simulink model "Wind1500KW_bilbil_finished"  (R2020a)
settings: Solver=VariableStepAuto  StartTime=0.0  StopTime=20  RelTol=1e-3
libraries: powerlib x12, powerlib_meascontrol x10, simulink x7
settings Model: Creator=Administrator  LastModifiedBy=Administrator

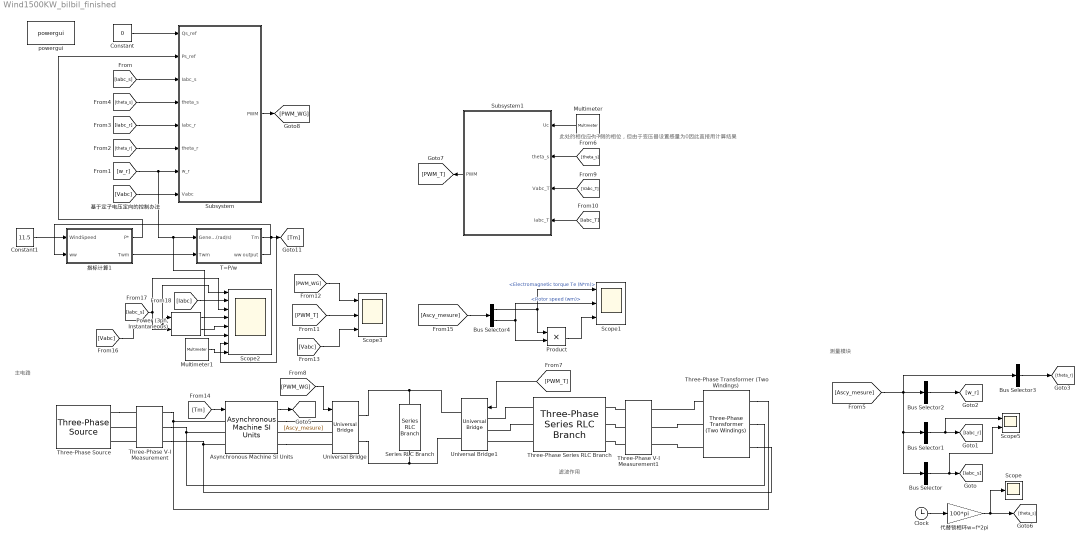
== system Wind1500KW_bilbil_finished ==
  note: 滤波作用
  note: 此处的相位应为T侧的相位，但由于变压器设置感量为0因此直接用计算结果
  note: 测量模块
  note: 主电路
  Asynchronous Machine SI Units : powerlib/Machines/Asynchronous Machine SI Units  RotorType=Wound  PresetModel=No  MechanicalLoad=Torque Tm  ShowDetailedParameters=on  ReferenceFrame=Rotor  Units=SI  MeasurementBus=off  NominalParameters=[1.5e+06 690 50]  Stator=[0.0055 1.56e-4]  Rotor=[0.00621 2.26e-04]  Cage1=[0.4155 0.002066]  Cage2=[0.4168 0.0003495]  Lm=0.01101  Mechanical=[30 0.005879 2]  PolePairs=2  InitialConditions=[0 0 0 0 0 0 0 0]  SimulateSaturation=off  Saturation=[14.03593122, 27.81365428, 53.79336849, 72.68890987, 97.98006896, 148.6815601, 215.7428561, 302.9841135, 428.7778367 ; 230, 322, 414, 460, 506, 552, 598, 644, 690]  LoadFlowParameters=1492000  TsPowergui=0  TsBlock=-1  IterativeModel=Trapezoidal non iterative  IterativeDiscreteModel=Trapezoidal non iterative  Pmec=1.492e+006
  Bus Selector : BusSelector  OutputSignals=Stator measurements.Stator current is_a (A),Stator measurements.Stator current is_b (A),Stator measurements.Stator current is_c (A)  OutputAsBus=on
  Bus Selector1 : BusSelector  OutputSignals=Rotor measurements.Rotor current ir_a (A),Rotor measurements.Rotor current ir_b (A),Rotor measurements.Rotor current ir_c (A)  OutputAsBus=on
  Bus Selector2 : BusSelector  OutputSignals=Mechanical.Rotor speed (wm)  OutputAsBus=on
  Bus Selector3 : BusSelector  OutputSignals=Mechanical.Rotor angle thetam (rad)  OutputAsBus=on
  Bus Selector4 : BusSelector  OutputSignals=Mechanical.Electromagnetic torque Te (N*m),Mechanical.Rotor speed (wm)
  Clock : Clock
  Constant : Constant  Value=0
  Constant1 : Constant  Value=11.5
  Multimeter : powerlib/Measurements/Multimeter  PhasorSimulation=off  OutputType=Complex  sel=1  L=1  Gain=1  yselected={'Ub: Series RLC Branch'};  PSBOutputType=1  PSBequivalent=0  AxesSetting=[0,0.1,-100,100]  Display=0  SavedBlockNames=-11
  Multimeter1 : powerlib/Measurements/Multimeter  PhasorSimulation=off  OutputType=Complex  sel=1  L=1  Gain=1  yselected={'Ub: Series RLC Branch'};  PSBOutputType=1  PSBequivalent=0  AxesSetting=[0,0.1,-100,100]  Display=0  SavedBlockNames=-11
  "Power (3ph, Instantaneous)" : powerlib_meascontrol/Measurements/Power (3ph, Instantaneous)
  Product : Product
  Scope : Scope
  Scope1 : Scope  NumInputPorts=3
  Scope2 : Scope  NumInputPorts=8
  Scope3 : Scope  NumInputPorts=3
  Scope5 : Scope  NumInputPorts=2
  Series RLC Branch : powerlib/Elements/Series RLC Branch  LConnTagsString=__new0  RConnTagsString=__new0  BranchType=C  Resistance=1  Inductance=1e-3  SetiL0=off  InitialCurrent=0  Capacitance=1e-2  Setx0=off  InitialVoltage=1200  Measurements=Branch voltage
  Subsystem : Subsystem
  Subsystem1 : Subsystem
  T=P/w : Subsystem
  Three-Phase Series RLC Branch : powerlib/Elements/Three-Phase Series RLC Branch  LConnTagsString=A|B|C  RConnTagsString=A|B|C  BranchType=RL  Resistance=0.05  Inductance=1.2e-2  Capacitance=1e-6  Measurements=None
  Three-Phase Transformer (Two Windings) : powerlib/Elements/Three-Phase Transformer (Two Windings)  Winding1Connection=Yg  Winding2Connection=Yg  CoreType=Three single-phase transformers  SetSaturation=off  Hysteresis=off  DataFile='hysteresis'  SetInitialFlux=off  Measurements=None  UNITS=SI  NominalPower=[ 1e6 , 50 ]  Winding1=[890 0.001 0]  Winding2=[690 0.001 0]  Rm=1.0805e+03  Lm=4  L0=0.5  Saturation=[0 0;0.66653 1910.3;277.72 2419.7]  InitialFluxes=[ 0.8 , -0.8 , 0.7 ]  BreakLoop=off  DiscreteSolver=Backward Euler robust  DataType=on  TransfoNumber=1
  Three-Phase V-I Measurement : powerlib/Measurements/Three-Phase V-I Measurement  VoltageMeasurement=phase-to-ground  SetLabelV=on  LabelV=Vabc  Vpu=off  VpuLL=off  CurrentMeasurement=yes  SetLabelI=on  LabelI=Iabc  Ipu=off  Pbase=100e6  Vbase=500e3  OutputType=Complex  PhasorSimulation=off  PSBequivalent=0
  Three-Phase V-I Measurement1 : powerlib/Measurements/Three-Phase V-I Measurement  VoltageMeasurement=phase-to-ground  SetLabelV=on  LabelV=Vabc_T  Vpu=off  VpuLL=off  CurrentMeasurement=yes  SetLabelI=on  LabelI=Iabc_T  Ipu=off  Pbase=100e6  Vbase=500e3  OutputType=Complex  PhasorSimulation=off  PSBequivalent=0
  Three-Phase Source : powerlib/Electrical Sources/Three-Phase Source  InternalConnection=Yg  VoltagePhases=off  Voltage=690  PhaseAngle=0  Voltage_phases=[25e3 25e3 25e3]/sqrt(3)  PhaseAngles_phases=[0 -120 +120]  Frequency=50  NonIdealSource=off  SpecifyImpedance=off  Resistance=0.8929  Inductance=16.58e-3  ShortCircuitLevel=100e6  BaseVoltage=690  XRratio=7  BusType=swing  Pref=10e3  Qref=0  Prefabc=[10e3, 10e3, 10e3]  Qrefabc=[0, 0, 0]  Qmin=-inf  Qmax=inf
  Universal Bridge : powerlib/Power Electronics/Universal Bridge  Arms=3  SnubberResistance=1e5  SnubberCapacitance=inf  Device=MOSFET / Diodes  Ron=1e-3  Lon=0  ForwardVoltages="[  0  0  ]"  ForwardVoltage=0  GTOparameters=[ 10e-6 , 20e-6 ]  IGBTparameters=[ 1e-6 , 2e-6 ]  Measurements=None  Measurements_2=None  converterType=Rectifier
  Universal Bridge1 : powerlib/Power Electronics/Universal Bridge  Arms=3  SnubberResistance=1e5  SnubberCapacitance=inf  Device=MOSFET / Diodes  Ron=1e-3  Lon=0  ForwardVoltages="[  0  0  ]"  ForwardVoltage=0  GTOparameters=[ 10e-6 , 20e-6 ]  IGBTparameters=[ 1e-6 , 2e-6 ]  Measurements=None  Measurements_2=None  converterType=Rectifier
  powergui : powerlib/powergui  Priority=1  SimulationMode=Discrete  SampleTime=5e-6  frequency=60  Iterations=50  frequencyindice=50  Pbase=100e6  ErrMax=1e-4  UnitsV=kV  UnitsW=MW  buscounter=0  FunctionMessages=off  echomessages=off  EnableUseOfTLC=off  CurrentSourceSwitches=off  DisableSnubberDevices=off  DisableRonSwitches=off  DisableVfSwitches=off  DisplayEquations=off  AutomaticDiscreteSolvers=off  SolverType=Tustin/Backward Euler (TBE)  Interpol=off  ExternalGateDelay=off  methode=off  Ts=100  x0status=blocks  SPID=on  SwTol=0  HookPort=off  NonlinearTolerance=1e-4  nMaxIteration=100  ContinueOnMaxIteration=off  RestoreLinks=warning  ResistiveCurrentMeasurement=off  Frange=[0:2:500]  Ylog=off  Xlog=on  ShowGrid=off  save=off  variable=ZData  structure=0  ZoomFFT=off  StartTime=0.0  cycles=1  DisplayStyle=1  fundamental=60  FreqAxis=off  MaxFrequency=1000  frequencyindicesteady=1  RmsSteady=1  display=off
  代替锁相环w=f*2pi : Gain  Gain=100*pi
  指标计算1 : Subsystem
  wires:
  指标计算1/2(Twm) -> T=P/w/2(Twm)
  T=P/w/2(ww output) -> 指标计算1/2(ww)
  Clock/1 -> 代替锁相环w=f*2pi/1
  代替锁相环w=f*2pi/1 -> [theta_s], Scope/1
  Bus Selector/1 -> Scope5/2, [Iabc_s]
  Bus Selector1/1 -> Scope5/1, [Iabc_r]
  Bus Selector2/1 -> [w_r]
  Bus Selector3/1 -> [theta_r]
  Bus Selector4/1 -> Product/1, Scope1/1  "<Electromagnetic torque Te (N*m)>"
  Product/1 -> Scope1/3
  Bus Selector4/2 -> Scope1/2, Product/2  "<Rotor speed (wm)>"
  指标计算1/1(P*) -> Subsystem/2(Ps_ref)
  Constant/1 -> Subsystem/1(Qs_ref)
  [Iabc_s] -> Subsystem/3(Iabc_s)
  [w_r] -> Subsystem/7(w_r), Scope2/6, T=P/w/1(Generator Speed(rad/s))
  [theta_r] -> Subsystem/6(theta_r)
  [Iabc_r] -> Subsystem/5(Iabc_r)
  Constant1/1 -> 指标计算1/1(WindSpeed)
  [Vabc] -> Subsystem/8(Vabc)
  Asynchronous Machine SI Units/1 -> [Ascy_mesure]
  [Ascy_mesure] -> Bus Selector3/1, Bus Selector1/1, Bus Selector/1, Bus Selector2/1
  [theta_s] -> Subsystem/4(theta_s)
  [theta_s] -> Subsystem1/2(theta_s)
  Multimeter/1 -> Subsystem1/1(Uc)
  Subsystem1/1(PWM) -> [PWM_T]
  [PWM_T] -> Universal Bridge1/1
  Subsystem/1(PWM) -> [PWM_WG]
  [PWM_WG] -> Universal Bridge/1
  [Vabc] -> Scope3/3
  [PWM_T] -> Scope3/2
  [PWM_WG] -> Scope3/1
  [Vabc_T] -> Subsystem1/3(Vabc_T)
  [Iabc_T] -> Subsystem1/4(Iabc_T)
  T=P/w/1(Tm) -> Scope2/7, [Tm]
  [Tm] -> Asynchronous Machine SI Units/1
  [Vabc] -> Scope2/1, "Power (3ph, Instantaneous)"/1
  [Iabc_s] -> "Power (3ph, Instantaneous)"/2, Scope2/3
  "Power (3ph, Instantaneous)"/1 -> Scope2/4
  "Power (3ph, Instantaneous)"/2 -> Scope2/5
  [Iabc] -> Scope2/2
  Multimeter1/1 -> Scope2/8
  [Ascy_mesure] -> Bus Selector4/1
  connections:
  Three-Phase Source/RConn1 -- Three-Phase V-I Measurement/LConn1
  Three-Phase V-I Measurement/LConn2 -- Three-Phase Source/RConn2
  Three-Phase V-I Measurement/RConn1 -- Three-Phase Transformer (Two Windings)/RConn1 -- Asynchronous Machine SI Units/LConn1
  Three-Phase V-I Measurement/RConn2 -- Three-Phase Transformer (Two Windings)/RConn2 -- Asynchronous Machine SI Units/LConn2
  Three-Phase V-I Measurement/RConn3 -- Three-Phase Transformer (Two Windings)/RConn3 -- Asynchronous Machine SI Units/LConn3
  Three-Phase V-I Measurement/LConn3 -- Three-Phase Source/RConn3
  Universal Bridge/LConn2 -- Asynchronous Machine SI Units/RConn2
  Asynchronous Machine SI Units/RConn1 -- Universal Bridge/LConn1
  Asynchronous Machine SI Units/RConn3 -- Universal Bridge/LConn3
  Universal Bridge/RConn1 -- Universal Bridge1/RConn1 -- Series RLC Branch/LConn1
  Universal Bridge/RConn2 -- Series RLC Branch/RConn1 -- Universal Bridge1/RConn2
  Three-Phase Series RLC Branch/LConn1 -- Universal Bridge1/LConn1
  Three-Phase Series RLC Branch/LConn2 -- Universal Bridge1/LConn2
  Three-Phase Series RLC Branch/LConn3 -- Universal Bridge1/LConn3
  Three-Phase V-I Measurement1/LConn1 -- Three-Phase Series RLC Branch/RConn1
  Three-Phase V-I Measurement1/LConn2 -- Three-Phase Series RLC Branch/RConn2
  Three-Phase V-I Measurement1/LConn3 -- Three-Phase Series RLC Branch/RConn3
  Three-Phase Transformer (Two Windings)/LConn2 -- Three-Phase V-I Measurement1/RConn2
  Three-Phase Transformer (Two Windings)/LConn1 -- Three-Phase V-I Measurement1/RConn1
  Three-Phase Transformer (Two Windings)/LConn3 -- Three-Phase V-I Measurement1/RConn3

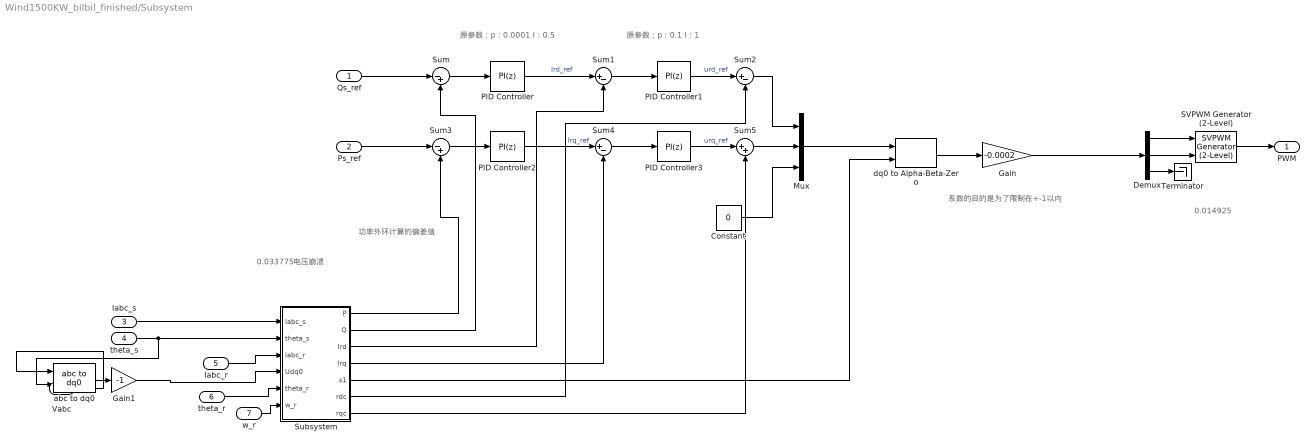
== system Wind1500KW_bilbil_finished/Subsystem ==
  note: 原参数：p：0.0001 I：0.5
  note: 0.033775电压崩溃
  note: 0.014925
  note: 系数的目的是为了限制在+-1以内
  note: 功率外环计算的偏差值
  note: 原参数：p：0.1 I：1
  Qs_ref : Inport
  Ps_ref : Inport  Port=2
  Iabc_s : Inport  Port=3
  theta_s : Inport  Port=4
  Iabc_r : Inport  Port=5
  theta_r : Inport  Port=6
  w_r : Inport  Port=7
  Vabc : Inport  Port=8
  Constant : Constant  Value=0
  Demux : Demux  Outputs=3
  Gain : Gain  Gain=-0.0002
  Gain1 : Gain  Gain=-1
  Mux : Mux  Inputs=3
  PID Controller : simulink/Continuous/PID Controller  Controller=PI  Form=Parallel  TimeDomain=Discrete-time  UseExternalTs=off  SampleTime=5e-6  IntegratorMethod=Forward Euler  FilterMethod=Forward Euler  ControllerParametersSource=internal  P=0.0001  I=0.5  D=0  UseFilter=on  N=100  TunerSelectOption=Transfer Function Based (PID Tuner App)  InitialConditionSource=internal  InitialConditionForIntegrator=0  InitialConditionForFilter=0  DifferentiatorICPrevScaledInput=0  ExternalReset=none  TrackingMode=off  Kt=1  LimitOutput=off  UpperSaturationLimit=inf  LowerSaturationLimit=-inf  LinearizeAsGain=on  AntiWindupMode=none  Kb=1  POutMin=[]  POutMax=[]  IOutMin=[]  IOutMax=[]  DOutMin=[]  DOutMax=[]  NOutMin=[]  NOutMax=[]  SumOutMin=[]  SumOutMax=[]  SaturationOutMin=[]  SaturationOutMax=[]  PParamMin=[]  PParamMax=[]  IParamMin=[]  IParamMax=[]  DParamMin=[]  DParamMax=[]  NParamMin=[]  NParamMax=[]  KbParamMin=[]  KbParamMax=[]  KtParamMin=[]  KtParamMax=[]  KbOutMin=[]  KbOutMax=[]  KtOutMin=[]  KtOutMax=[]  IntegratorOutMin=[]  IntegratorOutMax=[]  FilterOutMin=[]  FilterOutMax=[]  SumI1OutMin=[]  SumI1OutMax=[]  SumI2OutMin=[]  SumI2OutMax=[]  SumI3OutMin=[]  SumI3OutMax=[]  SumI4OutMin=[]  SumI4OutMax=[]  SumDOutMin=[]  SumDOutMax=[]  DifferentiatorOutMin=[]  DifferentiatorOutMax=[]  FilterDiffOutCoefMin=[]  FilterDiffOutCoefMax=[]  ReciprocalOutMin=[]  ReciprocalOutMax=[]  SumDenOutMin=[]  SumDenOutMax=[]  SumNumOutMin=[]  SumNumOutMax=[]  DivideOutMin=[]  DivideOutMax=[]  UdiffTsProdOutMin=[]  UdiffTsProdOutMax=[]  NTsProdOutMin=[]  NTsProdOutMax=[]  UintegralTsProdOutMin=[]  UintegralTsProdOutMax=[]  UngainTsProdOutMin=[]  UngainTsProdOutMax=[]  IntegratorContinuousStateAttributes=''  IntegratorStateMustResolveToSignalObject=off  IntegratorRTWStateStorageClass=Auto  FilterContinuousStateAttributes=''  FilterStateMustResolveToSignalObject=off  FilterRTWStateStorageClass=Auto  ParallelPVariant=InternalParameters  IdealPVariant=Disabled  IVariant=InternalParameters  DVariant=Disabled  IntegratorVariant=Discrete  SatVariant=Disabled  AWVariant=Passthrough  PCopyVariant=Disabled  TRVariant=Disabled  FdbkBlocksVariant=Forward  IdealPFdbkVariant=Disabled  SatFdbkVariant=Disabled  DerivativeFilterVariant=Disabled  NVariant=Disabled  NCopyVariant=Disabled_SignalSpec  FilterICVariant=Disabled  IntegratorICVariant=InternalICs  ExternalResetVariant=Disabled  TRSumVariant=Passthrough  SumFdbkVariant=Disabled  SumVariant=Sum_PI  TsampFilterVariant=InternalTs  TsampNgainVariant=Passthrough  TsampIntegralVariant=Passthrough
  PID Controller1 : simulink/Continuous/PID Controller  Controller=PI  Form=Parallel  TimeDomain=Discrete-time  UseExternalTs=off  SampleTime=5e-6  IntegratorMethod=Forward Euler  FilterMethod=Forward Euler  ControllerParametersSource=internal  P=0.1  I=1.3  D=0  UseFilter=on  N=100  TunerSelectOption=Transfer Function Based (PID Tuner App)  InitialConditionSource=internal  InitialConditionForIntegrator=0  InitialConditionForFilter=0  DifferentiatorICPrevScaledInput=0  ExternalReset=none  TrackingMode=off  Kt=1  LimitOutput=off  UpperSaturationLimit=inf  LowerSaturationLimit=-inf  LinearizeAsGain=on  AntiWindupMode=none  Kb=1  POutMin=[]  POutMax=[]  IOutMin=[]  IOutMax=[]  DOutMin=[]  DOutMax=[]  NOutMin=[]  NOutMax=[]  SumOutMin=[]  SumOutMax=[]  SaturationOutMin=[]  SaturationOutMax=[]  PParamMin=[]  PParamMax=[]  IParamMin=[]  IParamMax=[]  DParamMin=[]  DParamMax=[]  NParamMin=[]  NParamMax=[]  KbParamMin=[]  KbParamMax=[]  KtParamMin=[]  KtParamMax=[]  KbOutMin=[]  KbOutMax=[]  KtOutMin=[]  KtOutMax=[]  IntegratorOutMin=[]  IntegratorOutMax=[]  FilterOutMin=[]  FilterOutMax=[]  SumI1OutMin=[]  SumI1OutMax=[]  SumI2OutMin=[]  SumI2OutMax=[]  SumI3OutMin=[]  SumI3OutMax=[]  SumI4OutMin=[]  SumI4OutMax=[]  SumDOutMin=[]  SumDOutMax=[]  DifferentiatorOutMin=[]  DifferentiatorOutMax=[]  FilterDiffOutCoefMin=[]  FilterDiffOutCoefMax=[]  ReciprocalOutMin=[]  ReciprocalOutMax=[]  SumDenOutMin=[]  SumDenOutMax=[]  SumNumOutMin=[]  SumNumOutMax=[]  DivideOutMin=[]  DivideOutMax=[]  UdiffTsProdOutMin=[]  UdiffTsProdOutMax=[]  NTsProdOutMin=[]  NTsProdOutMax=[]  UintegralTsProdOutMin=[]  UintegralTsProdOutMax=[]  UngainTsProdOutMin=[]  UngainTsProdOutMax=[]  IntegratorContinuousStateAttributes=''  IntegratorStateMustResolveToSignalObject=off  IntegratorRTWStateStorageClass=Auto  FilterContinuousStateAttributes=''  FilterStateMustResolveToSignalObject=off  FilterRTWStateStorageClass=Auto  ParallelPVariant=InternalParameters  IdealPVariant=Disabled  IVariant=InternalParameters  DVariant=Disabled  IntegratorVariant=Discrete  SatVariant=Disabled  AWVariant=Passthrough  PCopyVariant=Disabled  TRVariant=Disabled  FdbkBlocksVariant=Forward  IdealPFdbkVariant=Disabled  SatFdbkVariant=Disabled  DerivativeFilterVariant=Disabled  NVariant=Disabled  NCopyVariant=Disabled_SignalSpec  FilterICVariant=Disabled  IntegratorICVariant=InternalICs  ExternalResetVariant=Disabled  TRSumVariant=Passthrough  SumFdbkVariant=Disabled  SumVariant=Sum_PI  TsampFilterVariant=InternalTs  TsampNgainVariant=Passthrough  TsampIntegralVariant=Passthrough
  PID Controller2 : simulink/Continuous/PID Controller  Controller=PI  Form=Parallel  TimeDomain=Discrete-time  UseExternalTs=off  SampleTime=5e-6  IntegratorMethod=Forward Euler  FilterMethod=Forward Euler  ControllerParametersSource=internal  P=0.0001  I=0.5  D=0  UseFilter=on  N=100  TunerSelectOption=Transfer Function Based (PID Tuner App)  InitialConditionSource=internal  InitialConditionForIntegrator=0  InitialConditionForFilter=0  DifferentiatorICPrevScaledInput=0  ExternalReset=none  TrackingMode=off  Kt=1  LimitOutput=off  UpperSaturationLimit=inf  LowerSaturationLimit=-inf  LinearizeAsGain=on  AntiWindupMode=none  Kb=1  POutMin=[]  POutMax=[]  IOutMin=[]  IOutMax=[]  DOutMin=[]  DOutMax=[]  NOutMin=[]  NOutMax=[]  SumOutMin=[]  SumOutMax=[]  SaturationOutMin=[]  SaturationOutMax=[]  PParamMin=[]  PParamMax=[]  IParamMin=[]  IParamMax=[]  DParamMin=[]  DParamMax=[]  NParamMin=[]  NParamMax=[]  KbParamMin=[]  KbParamMax=[]  KtParamMin=[]  KtParamMax=[]  KbOutMin=[]  KbOutMax=[]  KtOutMin=[]  KtOutMax=[]  IntegratorOutMin=[]  IntegratorOutMax=[]  FilterOutMin=[]  FilterOutMax=[]  SumI1OutMin=[]  SumI1OutMax=[]  SumI2OutMin=[]  SumI2OutMax=[]  SumI3OutMin=[]  SumI3OutMax=[]  SumI4OutMin=[]  SumI4OutMax=[]  SumDOutMin=[]  SumDOutMax=[]  DifferentiatorOutMin=[]  DifferentiatorOutMax=[]  FilterDiffOutCoefMin=[]  FilterDiffOutCoefMax=[]  ReciprocalOutMin=[]  ReciprocalOutMax=[]  SumDenOutMin=[]  SumDenOutMax=[]  SumNumOutMin=[]  SumNumOutMax=[]  DivideOutMin=[]  DivideOutMax=[]  UdiffTsProdOutMin=[]  UdiffTsProdOutMax=[]  NTsProdOutMin=[]  NTsProdOutMax=[]  UintegralTsProdOutMin=[]  UintegralTsProdOutMax=[]  UngainTsProdOutMin=[]  UngainTsProdOutMax=[]  IntegratorContinuousStateAttributes=''  IntegratorStateMustResolveToSignalObject=off  IntegratorRTWStateStorageClass=Auto  FilterContinuousStateAttributes=''  FilterStateMustResolveToSignalObject=off  FilterRTWStateStorageClass=Auto  ParallelPVariant=InternalParameters  IdealPVariant=Disabled  IVariant=InternalParameters  DVariant=Disabled  IntegratorVariant=Discrete  SatVariant=Disabled  AWVariant=Passthrough  PCopyVariant=Disabled  TRVariant=Disabled  FdbkBlocksVariant=Forward  IdealPFdbkVariant=Disabled  SatFdbkVariant=Disabled  DerivativeFilterVariant=Disabled  NVariant=Disabled  NCopyVariant=Disabled_SignalSpec  FilterICVariant=Disabled  IntegratorICVariant=InternalICs  ExternalResetVariant=Disabled  TRSumVariant=Passthrough  SumFdbkVariant=Disabled  SumVariant=Sum_PI  TsampFilterVariant=InternalTs  TsampNgainVariant=Passthrough  TsampIntegralVariant=Passthrough
  PID Controller3 : simulink/Continuous/PID Controller  Controller=PI  Form=Parallel  TimeDomain=Discrete-time  UseExternalTs=off  SampleTime=5e-6  IntegratorMethod=Forward Euler  FilterMethod=Forward Euler  ControllerParametersSource=internal  P=0.1  I=1.3  D=0  UseFilter=on  N=100  TunerSelectOption=Transfer Function Based (PID Tuner App)  InitialConditionSource=internal  InitialConditionForIntegrator=0  InitialConditionForFilter=0  DifferentiatorICPrevScaledInput=0  ExternalReset=none  TrackingMode=off  Kt=1  LimitOutput=off  UpperSaturationLimit=inf  LowerSaturationLimit=-inf  LinearizeAsGain=on  AntiWindupMode=none  Kb=1  POutMin=[]  POutMax=[]  IOutMin=[]  IOutMax=[]  DOutMin=[]  DOutMax=[]  NOutMin=[]  NOutMax=[]  SumOutMin=[]  SumOutMax=[]  SaturationOutMin=[]  SaturationOutMax=[]  PParamMin=[]  PParamMax=[]  IParamMin=[]  IParamMax=[]  DParamMin=[]  DParamMax=[]  NParamMin=[]  NParamMax=[]  KbParamMin=[]  KbParamMax=[]  KtParamMin=[]  KtParamMax=[]  KbOutMin=[]  KbOutMax=[]  KtOutMin=[]  KtOutMax=[]  IntegratorOutMin=[]  IntegratorOutMax=[]  FilterOutMin=[]  FilterOutMax=[]  SumI1OutMin=[]  SumI1OutMax=[]  SumI2OutMin=[]  SumI2OutMax=[]  SumI3OutMin=[]  SumI3OutMax=[]  SumI4OutMin=[]  SumI4OutMax=[]  SumDOutMin=[]  SumDOutMax=[]  DifferentiatorOutMin=[]  DifferentiatorOutMax=[]  FilterDiffOutCoefMin=[]  FilterDiffOutCoefMax=[]  ReciprocalOutMin=[]  ReciprocalOutMax=[]  SumDenOutMin=[]  SumDenOutMax=[]  SumNumOutMin=[]  SumNumOutMax=[]  DivideOutMin=[]  DivideOutMax=[]  UdiffTsProdOutMin=[]  UdiffTsProdOutMax=[]  NTsProdOutMin=[]  NTsProdOutMax=[]  UintegralTsProdOutMin=[]  UintegralTsProdOutMax=[]  UngainTsProdOutMin=[]  UngainTsProdOutMax=[]  IntegratorContinuousStateAttributes=''  IntegratorStateMustResolveToSignalObject=off  IntegratorRTWStateStorageClass=Auto  FilterContinuousStateAttributes=''  FilterStateMustResolveToSignalObject=off  FilterRTWStateStorageClass=Auto  ParallelPVariant=InternalParameters  IdealPVariant=Disabled  IVariant=InternalParameters  DVariant=Disabled  IntegratorVariant=Discrete  SatVariant=Disabled  AWVariant=Passthrough  PCopyVariant=Disabled  TRVariant=Disabled  FdbkBlocksVariant=Forward  IdealPFdbkVariant=Disabled  SatFdbkVariant=Disabled  DerivativeFilterVariant=Disabled  NVariant=Disabled  NCopyVariant=Disabled_SignalSpec  FilterICVariant=Disabled  IntegratorICVariant=InternalICs  ExternalResetVariant=Disabled  TRSumVariant=Passthrough  SumFdbkVariant=Disabled  SumVariant=Sum_PI  TsampFilterVariant=InternalTs  TsampNgainVariant=Passthrough  TsampIntegralVariant=Passthrough
  SVPWM Generator (2-Level) : powerlib_meascontrol/Pulse & Signal Generators/SVPWM Generator (2-Level)  InputType=alpha-beta components  SwitchingPattern=Pattern #1  Fc=3000  ParUref=[0.8 -30 50]  Ts=0
      settings: SourceProductBaseCode=PS
  Subsystem : Subsystem
  Sum : Sum  Inputs=|-+
  Sum1 : Sum  Inputs=|+-
  Sum2 : Sum  Inputs=|+-
  Sum3 : Sum  Inputs=|-+
  Sum4 : Sum  Inputs=|+-
  Sum5 : Sum  Inputs=|++
  Terminator : Terminator
  abc to dq0 : powerlib_meascontrol/Transformations/abc to dq0  Alignment=Aligned with phase A axis
  dq0 to Alpha-Beta-Zero : powerlib_meascontrol/Transformations/dq0 to Alpha-Beta-Zero  Alignment=Aligned with phase A axis
      settings: SourceProductBaseCode=PS
  PWM : Outport
  wires:
  Qs_ref/1 -> Sum/1
  Sum/1 -> PID Controller/1
  PID Controller/1 -> Sum1/1  "Ird_ref"
  Sum1/1 -> PID Controller1/1
  PID Controller1/1 -> Sum2/1  "urd_ref"
  Sum4/1 -> PID Controller3/1
  PID Controller3/1 -> Sum5/1  "urq_ref"
  PID Controller2/1 -> Sum4/1  "Irq_ref"
  Sum3/1 -> PID Controller2/1
  Ps_ref/1 -> Sum3/1
  Sum2/1 -> Mux/1
  Sum5/1 -> Mux/2
  Constant/1 -> Mux/3
  Mux/1 -> dq0 to Alpha-Beta-Zero/1
  dq0 to Alpha-Beta-Zero/1 -> Gain/1
  Demux/1 -> SVPWM Generator (2-Level)/1
  Demux/2 -> SVPWM Generator (2-Level)/2
  Demux/3 -> Terminator/1
  SVPWM Generator (2-Level)/1 -> PWM/1
  Vabc/1 -> abc to dq0/1
  theta_s/1 -> Subsystem/2(theta_s), abc to dq0/2
  abc to dq0/1 -> Gain1/1
  Subsystem/3(Ird) -> Sum1/2
  Subsystem/4(Irq) -> Sum4/2
  Subsystem/1(P) -> Sum3/2
  Subsystem/7(rqc) -> Sum5/2
  Subsystem/6(rdc) -> Sum2/2
  Subsystem/5(s1) -> dq0 to Alpha-Beta-Zero/2
  Subsystem/2(Q) -> Sum/2
  Gain/1 -> Demux/1
  Iabc_s/1 -> Subsystem/1(Iabc_s)
  Iabc_r/1 -> Subsystem/3(Iabc_r)
  theta_r/1 -> Subsystem/5(theta_r)
  w_r/1 -> Subsystem/6(w_r)
  Gain1/1 -> Subsystem/4(Udq0)

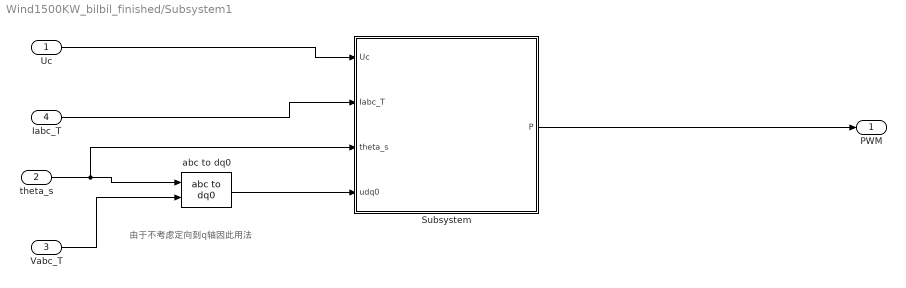
== system Wind1500KW_bilbil_finished/Subsystem1 ==
  note: 由于不考虑定向到q轴因此用法
  Uc : Inport
  theta_s : Inport  Port=2
  Vabc_T : Inport  Port=3
  Iabc_T : Inport  Port=4
  Subsystem : Subsystem
  abc to dq0 : powerlib_meascontrol/Transformations/abc to dq0  Alignment=90 degrees behind phase A axis
  PWM : Outport
  wires:
  Vabc_T/1 -> abc to dq0/1
  theta_s/1 -> abc to dq0/2, Subsystem/3(theta_s)
  Uc/1 -> Subsystem/1(Uc)
  Iabc_T/1 -> Subsystem/2(Iabc_T)
  abc to dq0/1 -> Subsystem/4(udq0)
  Subsystem/1(P) -> PWM/1

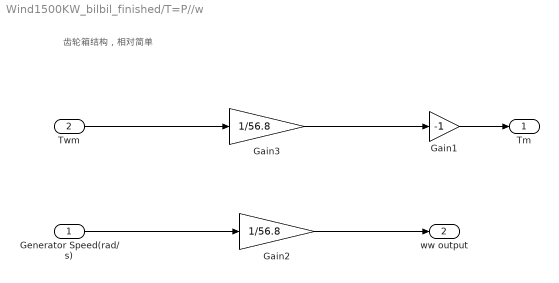
== system Wind1500KW_bilbil_finished/T=P//w ==
  note: 齿轮箱结构，相对简单
  Generator Speed(rad/s) : Inport
  Twm : Inport  Port=2
  Gain1 : Gain  Gain=-1
  Gain2 : Gain  Gain=1/56.8
  Gain3 : Gain  Gain=1/56.8
  Tm : Outport
  ww output : Outport  Port=2
  wires:
  Gain1/1 -> Tm/1
  Generator Speed(rad/s)/1 -> Gain2/1
  Gain2/1 -> ww output/1
  Twm/1 -> Gain3/1
  Gain3/1 -> Gain1/1

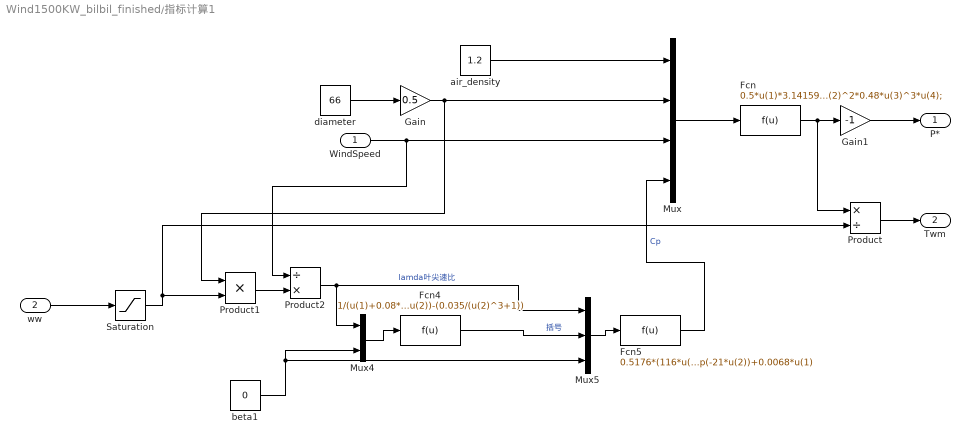
== system Wind1500KW_bilbil_finished/指标计算1 ==
  WindSpeed : Inport
  ww : Inport  Port=2
  Fcn : Fcn  Expr=0.5*u(1)*3.1415926*u(2)^2*0.48*u(3)^3*u(4);
  Fcn4 : Fcn  Expr=1/(u(1)+0.08*u(2))-(0.035/(u(2)^3+1))
  Fcn5 : Fcn  Expr=0.5176*(116*u(2)-0.4*u(3)-5)*exp(-21*u(2))+0.0068*u(1)
  Gain : Gain  Gain=0.5
  Gain1 : Gain  Gain=-1
  Mux : Mux
  Mux4 : Mux  Inputs=2
  Mux5 : Mux  Inputs=3
  Product : Product  Inputs=*/
  Product1 : Product
  Product2 : Product  Inputs=/*
  Saturation : Saturate  UpperLimit=1e6  LowerLimit=1e-6
  air_density : Constant  Value=1.2
  beta1 : Constant  Value=0
  diameter : Constant  Value=66
  P* : Outport
  Twm : Outport  Port=2
  wires:
  Fcn/1 -> Product/1, Gain1/1
  WindSpeed/1 -> Product2/1, Mux/3
  Gain/1 -> Product1/1, Mux/2
  Mux/1 -> Fcn/1
  diameter/1 -> Gain/1
  air_density/1 -> Mux/1
  Gain1/1 -> P*/1
  ww/1 -> Saturation/1
  Product/1 -> Twm/1
  Saturation/1 -> Product/2, Product1/2
  Product1/1 -> Product2/2
  Product2/1 -> Mux5/1, Mux4/1  "lamda叶尖速比"
  Mux4/1 -> Fcn4/1
  Fcn4/1 -> Mux5/2  "括号"
  Mux5/1 -> Fcn5/1
  Fcn5/1 -> Mux/4  "Cp"
  beta1/1 -> Mux5/3, Mux4/2

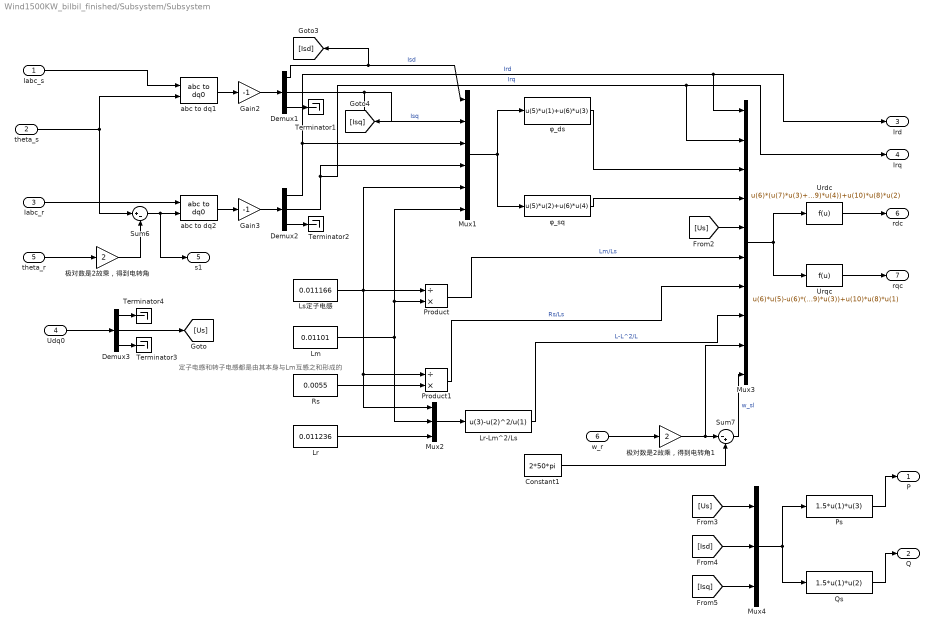
== system Wind1500KW_bilbil_finished/Subsystem/Subsystem ==
  note: 定子电感和转子电感都是由其本身与Lm互感之和形成的
  Iabc_s : Inport
  theta_s : Inport  Port=2
  Iabc_r : Inport  Port=3
  Udq0 : Inport  Port=4
  theta_r : Inport  Port=5
  w_r : Inport  Port=6
  Constant1 : Constant  Value=2*50*pi
  Demux1 : Demux  Outputs=3
  Demux2 : Demux  Outputs=3
  Demux3 : Demux  Outputs=3
  Gain2 : Gain  Gain=-1
  Gain3 : Gain  Gain=-1
  Lm : Constant  Value=0.01101
  Lr : Constant  Value=0.011236
  Lr-Lm^2/Ls : Fcn  Expr=u(3)-u(2)^2/u(1)
  Ls定子电感 : Constant  Value=0.011166
  Mux1 : Mux  Inputs=6
  Mux2 : Mux  Inputs=3
  Mux3 : Mux  Inputs=10
  Mux4 : Mux  Inputs=3
  Product : Product  Inputs=/*
  Product1 : Product  Inputs=/*
  Ps : Fcn  Expr=1.5*u(1)*u(3)
  Qs : Fcn  Expr=1.5*u(1)*u(2)
  Rs : Constant  Value=0.0055
  Sum6 : Sum  Inputs=|+-
  Sum7 : Sum  Inputs=|-+
  Terminator{1..4} (4 alike) : Terminator
  Urdc : Fcn  Expr=u(6)*(u(7)*u(3)+u(9)*u(4))+u(10)*u(8)*u(2)
  Urqc : Fcn  Expr=u(6)*u(5)-u(6)*(u(7)*u(4)+u(9)*u(3))+u(10)*u(8)*u(1)
  abc to dq1 : powerlib_meascontrol/Transformations/abc to dq0  Alignment=Aligned with phase A axis
  abc to dq2 : powerlib_meascontrol/Transformations/abc to dq0  Alignment=Aligned with phase A axis
  φ_ds : Fcn  Expr=u(5)*u(1)+u(6)*u(3)
  φ_sq : Fcn  Expr=u(5)*u(2)+u(6)*u(4)
  极对数是2故乘，得到电转角 : Gain  Gain=2
  极对数是2故乘，得到电转角1 : Gain  Gain=2
  P : Outport
  Q : Outport  Port=2
  Ird : Outport  Port=3
  Irq : Outport  Port=4
  s1 : Outport  Port=5
  rdc : Outport  Port=6
  rqc : Outport  Port=7
  wires:
  Ps/1 -> P/1
  Ls定子电感/1 -> Product1/1, Mux2/1, Product/1, Mux1/5
  Demux3/1 -> Terminator4/1
  Mux1/1 -> φ_sq/1, φ_ds/1
  Demux3/2 -> [Us]
  Demux1/2 -> [Isq], Mux1/2  "Isq"
  Gain3/1 -> Demux2/1
  Demux2/1 -> Mux3/1, Ird/1, Mux1/3  "Ird"
  Sum6/1 -> s1/1, abc to dq2/2
  Demux1/1 -> Mux1/1, [Isd]  "Isd"
  Qs/1 -> Q/1
  Demux2/2 -> Mux3/2, Irq/1, Mux1/4  "Irq"
  Lm/1 -> Mux2/2, Mux1/6, Product/2
  Demux2/3 -> Terminator2/1
  Mux3/1 -> Urqc/1, Urdc/1
  Rs/1 -> Product1/2
  Lr/1 -> Mux2/3
  Mux2/1 -> Lr-Lm^2/Ls/1
  Demux3/3 -> Terminator3/1
  Mux4/1 -> Qs/1, Ps/1
  φ_sq/1 -> Mux3/4
  极对数是2故乘，得到电转角1/1 -> Mux3/9, Sum7/1
  w_r/1 -> 极对数是2故乘，得到电转角1/1
  Demux1/3 -> Terminator1/1
  Gain2/1 -> Demux1/1
  abc to dq2/1 -> Gain3/1
  φ_ds/1 -> Mux3/3
  极对数是2故乘，得到电转角/1 -> Sum6/2
  [Isq] -> Mux4/3
  Product/1 -> Mux3/6  "Lm/Ls"
  [Us] -> Mux4/1
  abc to dq1/1 -> Gain2/1
  Product1/1 -> Mux3/7  "Rs/Ls"
  Constant1/1 -> Sum7/2
  Lr-Lm^2/Ls/1 -> Mux3/8  "L-L^2/L"
  [Isd] -> Mux4/2
  Iabc_r/1 -> abc to dq2/1
  Iabc_s/1 -> abc to dq1/1
  Urdc/1 -> rdc/1
  Udq0/1 -> Demux3/1
  Urqc/1 -> rqc/1
  theta_r/1 -> 极对数是2故乘，得到电转角/1
  theta_s/1 -> abc to dq1/2, Sum6/1
  Sum7/1 -> Mux3/10  "w_sl"
  [Us] -> Mux3/5

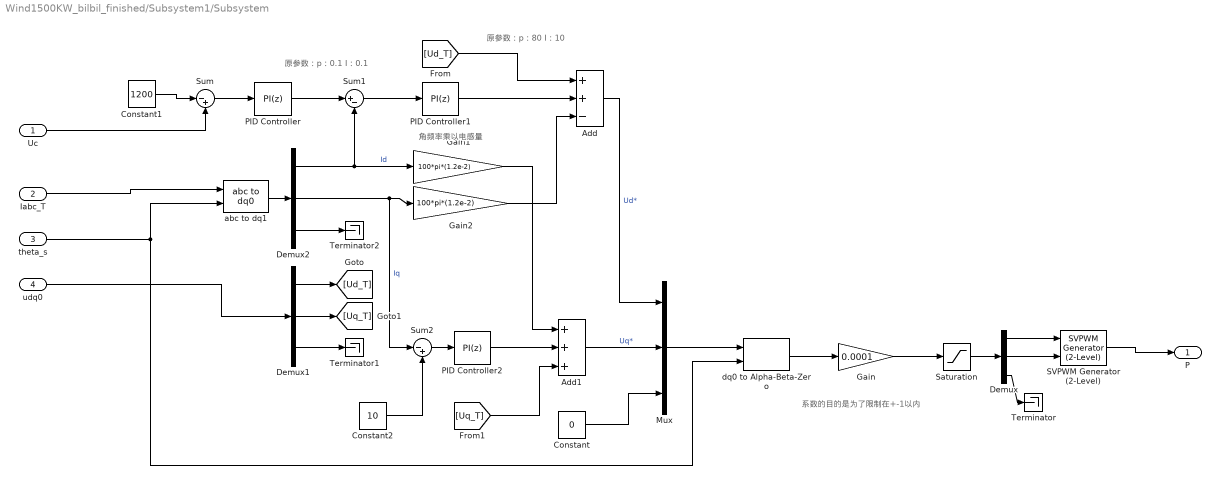
== system Wind1500KW_bilbil_finished/Subsystem1/Subsystem ==
  note: 角频率乘以电感量
  note: 系数的目的是为了限制在+-1以内
  note: 原参数：p：0.1 I：0.1
  note: 原参数：p：80 I：10
  Uc : Inport
  Iabc_T : Inport  Port=2
  theta_s : Inport  Port=3
  udq0 : Inport  Port=4
  Add : Sum  Inputs=++-
  Add1 : Sum  Inputs=+++
  Constant : Constant  Value=0
  Constant1 : Constant  Value=1200
  Constant2 : Constant  Value=10
  Demux : Demux  Outputs=3
  Demux1 : Demux  Outputs=3
  Demux2 : Demux  Outputs=3
  Gain : Gain  Gain=0.0001
  Gain1 : Gain  Gain=100*pi*(1.2e-2)
  Gain2 : Gain  Gain=100*pi*(1.2e-2)
  Mux : Mux  Inputs=3
  PID Controller : simulink/Continuous/PID Controller  Controller=PI  Form=Parallel  TimeDomain=Discrete-time  UseExternalTs=off  SampleTime=5e-6  IntegratorMethod=Forward Euler  FilterMethod=Forward Euler  ControllerParametersSource=internal  P=2  I=0.1  D=0  UseFilter=on  N=100  TunerSelectOption=Transfer Function Based (PID Tuner App)  InitialConditionSource=internal  InitialConditionForIntegrator=0  InitialConditionForFilter=0  DifferentiatorICPrevScaledInput=0  ExternalReset=none  TrackingMode=off  Kt=1  LimitOutput=off  UpperSaturationLimit=inf  LowerSaturationLimit=-inf  LinearizeAsGain=on  AntiWindupMode=none  Kb=1  POutMin=[]  POutMax=[]  IOutMin=[]  IOutMax=[]  DOutMin=[]  DOutMax=[]  NOutMin=[]  NOutMax=[]  SumOutMin=[]  SumOutMax=[]  SaturationOutMin=[]  SaturationOutMax=[]  PParamMin=[]  PParamMax=[]  IParamMin=[]  IParamMax=[]  DParamMin=[]  DParamMax=[]  NParamMin=[]  NParamMax=[]  KbParamMin=[]  KbParamMax=[]  KtParamMin=[]  KtParamMax=[]  KbOutMin=[]  KbOutMax=[]  KtOutMin=[]  KtOutMax=[]  IntegratorOutMin=[]  IntegratorOutMax=[]  FilterOutMin=[]  FilterOutMax=[]  SumI1OutMin=[]  SumI1OutMax=[]  SumI2OutMin=[]  SumI2OutMax=[]  SumI3OutMin=[]  SumI3OutMax=[]  SumI4OutMin=[]  SumI4OutMax=[]  SumDOutMin=[]  SumDOutMax=[]  DifferentiatorOutMin=[]  DifferentiatorOutMax=[]  FilterDiffOutCoefMin=[]  FilterDiffOutCoefMax=[]  ReciprocalOutMin=[]  ReciprocalOutMax=[]  SumDenOutMin=[]  SumDenOutMax=[]  SumNumOutMin=[]  SumNumOutMax=[]  DivideOutMin=[]  DivideOutMax=[]  UdiffTsProdOutMin=[]  UdiffTsProdOutMax=[]  NTsProdOutMin=[]  NTsProdOutMax=[]  UintegralTsProdOutMin=[]  UintegralTsProdOutMax=[]  UngainTsProdOutMin=[]  UngainTsProdOutMax=[]  IntegratorContinuousStateAttributes=''  IntegratorStateMustResolveToSignalObject=off  IntegratorRTWStateStorageClass=Auto  FilterContinuousStateAttributes=''  FilterStateMustResolveToSignalObject=off  FilterRTWStateStorageClass=Auto  ParallelPVariant=InternalParameters  IdealPVariant=Disabled  IVariant=InternalParameters  DVariant=Disabled  IntegratorVariant=Discrete  SatVariant=Disabled  AWVariant=Passthrough  PCopyVariant=Disabled  TRVariant=Disabled  FdbkBlocksVariant=Forward  IdealPFdbkVariant=Disabled  SatFdbkVariant=Disabled  DerivativeFilterVariant=Disabled  NVariant=Disabled  NCopyVariant=Disabled_SignalSpec  FilterICVariant=Disabled  IntegratorICVariant=InternalICs  ExternalResetVariant=Disabled  TRSumVariant=Passthrough  SumFdbkVariant=Disabled  SumVariant=Sum_PI  TsampFilterVariant=InternalTs  TsampNgainVariant=Passthrough  TsampIntegralVariant=Passthrough
  PID Controller1 : simulink/Continuous/PID Controller  Controller=PI  Form=Parallel  TimeDomain=Discrete-time  UseExternalTs=off  SampleTime=5e-6  IntegratorMethod=Forward Euler  FilterMethod=Forward Euler  ControllerParametersSource=internal  P=80  I=10  D=0  UseFilter=on  N=100  TunerSelectOption=Transfer Function Based (PID Tuner App)  InitialConditionSource=internal  InitialConditionForIntegrator=0  InitialConditionForFilter=0  DifferentiatorICPrevScaledInput=0  ExternalReset=none  TrackingMode=off  Kt=1  LimitOutput=off  UpperSaturationLimit=inf  LowerSaturationLimit=-inf  LinearizeAsGain=on  AntiWindupMode=none  Kb=1  POutMin=[]  POutMax=[]  IOutMin=[]  IOutMax=[]  DOutMin=[]  DOutMax=[]  NOutMin=[]  NOutMax=[]  SumOutMin=[]  SumOutMax=[]  SaturationOutMin=[]  SaturationOutMax=[]  PParamMin=[]  PParamMax=[]  IParamMin=[]  IParamMax=[]  DParamMin=[]  DParamMax=[]  NParamMin=[]  NParamMax=[]  KbParamMin=[]  KbParamMax=[]  KtParamMin=[]  KtParamMax=[]  KbOutMin=[]  KbOutMax=[]  KtOutMin=[]  KtOutMax=[]  IntegratorOutMin=[]  IntegratorOutMax=[]  FilterOutMin=[]  FilterOutMax=[]  SumI1OutMin=[]  SumI1OutMax=[]  SumI2OutMin=[]  SumI2OutMax=[]  SumI3OutMin=[]  SumI3OutMax=[]  SumI4OutMin=[]  SumI4OutMax=[]  SumDOutMin=[]  SumDOutMax=[]  DifferentiatorOutMin=[]  DifferentiatorOutMax=[]  FilterDiffOutCoefMin=[]  FilterDiffOutCoefMax=[]  ReciprocalOutMin=[]  ReciprocalOutMax=[]  SumDenOutMin=[]  SumDenOutMax=[]  SumNumOutMin=[]  SumNumOutMax=[]  DivideOutMin=[]  DivideOutMax=[]  UdiffTsProdOutMin=[]  UdiffTsProdOutMax=[]  NTsProdOutMin=[]  NTsProdOutMax=[]  UintegralTsProdOutMin=[]  UintegralTsProdOutMax=[]  UngainTsProdOutMin=[]  UngainTsProdOutMax=[]  IntegratorContinuousStateAttributes=''  IntegratorStateMustResolveToSignalObject=off  IntegratorRTWStateStorageClass=Auto  FilterContinuousStateAttributes=''  FilterStateMustResolveToSignalObject=off  FilterRTWStateStorageClass=Auto  ParallelPVariant=InternalParameters  IdealPVariant=Disabled  IVariant=InternalParameters  DVariant=Disabled  IntegratorVariant=Discrete  SatVariant=Disabled  AWVariant=Passthrough  PCopyVariant=Disabled  TRVariant=Disabled  FdbkBlocksVariant=Forward  IdealPFdbkVariant=Disabled  SatFdbkVariant=Disabled  DerivativeFilterVariant=Disabled  NVariant=Disabled  NCopyVariant=Disabled_SignalSpec  FilterICVariant=Disabled  IntegratorICVariant=InternalICs  ExternalResetVariant=Disabled  TRSumVariant=Passthrough  SumFdbkVariant=Disabled  SumVariant=Sum_PI  TsampFilterVariant=InternalTs  TsampNgainVariant=Passthrough  TsampIntegralVariant=Passthrough
  PID Controller2 : simulink/Continuous/PID Controller  Controller=PI  Form=Parallel  TimeDomain=Discrete-time  UseExternalTs=off  SampleTime=5e-6  IntegratorMethod=Forward Euler  FilterMethod=Forward Euler  ControllerParametersSource=internal  P=80  I=10  D=0  UseFilter=on  N=100  TunerSelectOption=Transfer Function Based (PID Tuner App)  InitialConditionSource=internal  InitialConditionForIntegrator=0  InitialConditionForFilter=0  DifferentiatorICPrevScaledInput=0  ExternalReset=none  TrackingMode=off  Kt=1  LimitOutput=off  UpperSaturationLimit=inf  LowerSaturationLimit=-inf  LinearizeAsGain=on  AntiWindupMode=none  Kb=1  POutMin=[]  POutMax=[]  IOutMin=[]  IOutMax=[]  DOutMin=[]  DOutMax=[]  NOutMin=[]  NOutMax=[]  SumOutMin=[]  SumOutMax=[]  SaturationOutMin=[]  SaturationOutMax=[]  PParamMin=[]  PParamMax=[]  IParamMin=[]  IParamMax=[]  DParamMin=[]  DParamMax=[]  NParamMin=[]  NParamMax=[]  KbParamMin=[]  KbParamMax=[]  KtParamMin=[]  KtParamMax=[]  KbOutMin=[]  KbOutMax=[]  KtOutMin=[]  KtOutMax=[]  IntegratorOutMin=[]  IntegratorOutMax=[]  FilterOutMin=[]  FilterOutMax=[]  SumI1OutMin=[]  SumI1OutMax=[]  SumI2OutMin=[]  SumI2OutMax=[]  SumI3OutMin=[]  SumI3OutMax=[]  SumI4OutMin=[]  SumI4OutMax=[]  SumDOutMin=[]  SumDOutMax=[]  DifferentiatorOutMin=[]  DifferentiatorOutMax=[]  FilterDiffOutCoefMin=[]  FilterDiffOutCoefMax=[]  ReciprocalOutMin=[]  ReciprocalOutMax=[]  SumDenOutMin=[]  SumDenOutMax=[]  SumNumOutMin=[]  SumNumOutMax=[]  DivideOutMin=[]  DivideOutMax=[]  UdiffTsProdOutMin=[]  UdiffTsProdOutMax=[]  NTsProdOutMin=[]  NTsProdOutMax=[]  UintegralTsProdOutMin=[]  UintegralTsProdOutMax=[]  UngainTsProdOutMin=[]  UngainTsProdOutMax=[]  IntegratorContinuousStateAttributes=''  IntegratorStateMustResolveToSignalObject=off  IntegratorRTWStateStorageClass=Auto  FilterContinuousStateAttributes=''  FilterStateMustResolveToSignalObject=off  FilterRTWStateStorageClass=Auto  ParallelPVariant=InternalParameters  IdealPVariant=Disabled  IVariant=InternalParameters  DVariant=Disabled  IntegratorVariant=Discrete  SatVariant=Disabled  AWVariant=Passthrough  PCopyVariant=Disabled  TRVariant=Disabled  FdbkBlocksVariant=Forward  IdealPFdbkVariant=Disabled  SatFdbkVariant=Disabled  DerivativeFilterVariant=Disabled  NVariant=Disabled  NCopyVariant=Disabled_SignalSpec  FilterICVariant=Disabled  IntegratorICVariant=InternalICs  ExternalResetVariant=Disabled  TRSumVariant=Passthrough  SumFdbkVariant=Disabled  SumVariant=Sum_PI  TsampFilterVariant=InternalTs  TsampNgainVariant=Passthrough  TsampIntegralVariant=Passthrough
  SVPWM Generator (2-Level) : powerlib_meascontrol/Pulse & Signal Generators/SVPWM Generator (2-Level)  InputType=alpha-beta components  SwitchingPattern=Pattern #1  Fc=2000  ParUref=[0.8 -30 50]  Ts=0
      settings: SourceProductBaseCode=PS
  Saturation : Saturate  UpperLimit=1  LowerLimit=-1
  Sum : Sum  Inputs=|-+
  Sum1 : Sum  Inputs=|+-
  Sum2 : Sum  Inputs=|-+
  Terminator : Terminator
  Terminator1 : Terminator
  Terminator2 : Terminator
  abc to dq1 : powerlib_meascontrol/Transformations/abc to dq0  Alignment=90 degrees behind phase A axis
  dq0 to Alpha-Beta-Zero : powerlib_meascontrol/Transformations/dq0 to Alpha-Beta-Zero  Alignment=90 degrees behind phase A axis
      settings: SourceProductBaseCode=PS
  P : Outport
  wires:
  Demux1/1 -> [Ud_T]
  theta_s/1 -> dq0 to Alpha-Beta-Zero/2, abc to dq1/2
  Demux/1 -> SVPWM Generator (2-Level)/1
  Sum2/1 -> PID Controller2/1
  SVPWM Generator (2-Level)/1 -> P/1
  Demux1/2 -> [Uq_T]
  Demux2/1 -> Gain1/1, Sum1/2  "Id"
  abc to dq1/1 -> Demux2/1
  [Uq_T] -> Add1/3
  Demux/2 -> SVPWM Generator (2-Level)/2
  Constant2/1 -> Sum2/2
  Constant1/1 -> Sum/1
  Gain/1 -> Saturation/1
  Demux2/3 -> Terminator2/1
  Gain2/1 -> Add/3
  Mux/1 -> dq0 to Alpha-Beta-Zero/1
  dq0 to Alpha-Beta-Zero/1 -> Gain/1
  Sum/1 -> PID Controller/1
  Add/1 -> Mux/1  "Ud*"
  PID Controller1/1 -> Add/2
  Demux2/2 -> Sum2/1, Gain2/1  "Iq"
  Sum1/1 -> PID Controller1/1
  Add1/1 -> Mux/2  "Uq*"
  Constant/1 -> Mux/3
  [Ud_T] -> Add/1
  Demux1/3 -> Terminator1/1
  PID Controller2/1 -> Add1/2
  Gain1/1 -> Add1/1
  Demux/3 -> Terminator/1
  PID Controller/1 -> Sum1/1
  udq0/1 -> Demux1/1
  Uc/1 -> Sum/2
  Iabc_T/1 -> abc to dq1/1
  Saturation/1 -> Demux/1
